simulink model "Area1"  (R2020a)
settings: Solver=VariableStepAuto  StartTime=0.0  StopTime=200  RelTol=1e-3
settings Model: Creator=prade  LastModifiedBy=prade

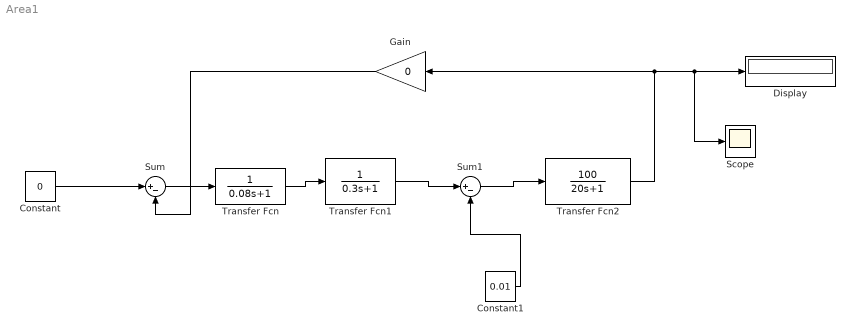
== system Area1 ==
  Constant : Constant  Value=0
  Constant1 : Constant  Value=0.01
  Display : Display
  Gain : Gain  Gain=0
  Scope : Scope
  Sum : Sum  Inputs=|+-
  Sum1 : Sum  Inputs=|+-
  Transfer Fcn : TransferFcn  Denominator=[0.08 1]
  Transfer Fcn1 : TransferFcn  Denominator=[0.3 1]
  Transfer Fcn2 : TransferFcn  Numerator=[100]  Denominator=[ 20 1]
  wires:
  Transfer Fcn2/1 -> Scope/1, Display/1, Gain/1
  Gain/1 -> Sum/2
  Sum/1 -> Transfer Fcn/1
  Transfer Fcn/1 -> Transfer Fcn1/1
  Constant/1 -> Sum/1
  Sum1/1 -> Transfer Fcn2/1
  Transfer Fcn1/1 -> Sum1/1
  Constant1/1 -> Sum1/2
